simulink model "bsm1_ss_singlereactor"  (R2012b)
settings: Solver=ode45  SolverMode=SingleTasking  StartTime=0.0  StopTime=14  FixedStep=0.01  RelTol=1e-5  AbsTol=1e-8
values from neighbouring files (symbols this model uses):
  ACTIVATE = [ 0 ]    [init_bsm1.m]
  carb1 = 0    [reginit_bsm1.m]    (also in reginit_bsm1_2.m)
  KLa1 = 2    [reginit_bsm1.m]    (also in reginit_bsm1_2.m)
  TEMPMODEL = [ 0 ]    [init_bsm1.m]
undefined symbols (not defined in the file or in its folder): PAR1, SOSAT1, VOL1, XINIT1
settings Model: ExtModeTrigMode=oneshot  ExtModeArmWhenConnect=off  ExtModeAutoUpdateStatusClock=off  BufferReuse=off  Creator=ielulf  LastModifiedBy=lasn
settings DataIOCC: InitialState=xFinal  LimitDataPoints=off  SignalLoggingSaveFormat=ModelDataLogs  SaveOutput=off  TimeSaveName=t  SignalLoggingName=sigsOut  OutputOption=SpecifiedOutputTimes  OutputTimes=[0:(1/96):14]
settings OptimizationCC: BlockReduction=off  BooleanDataType=off  InlineInvariantSignals=on  OptimizeBlockIOStorage=off  BufferReuse=off  ExpressionFolding=off  LocalBlockOutputs=off  InitFltsAndDblsToZero=on
settings DebuggingCC: SaveWithParameterizedLinksMsg=none  SignalResolutionControl=TryResolveAllWithWarning  SolverPrmCheckMsg=none  InheritedTsInSrcMsg=none  MultiTaskDSMMsg=warning  MultiTaskCondExecSysMsg=none  FcnCallInpInsideContextMsg=UseLocalSettings  UnconnectedOutputMsg=none  StrictBusMsg=None
settings HardwareCC: TargetUnknown=on
settings RTWCC: TemplateMakefile=grt_unix.tmf  IncludeERTFirstTime=on
settings GRTTargetCC: TargetFcnLib=ansi_tfl_tmw.mat  CombineOutputUpdateFcns=off  GRTInterface=on

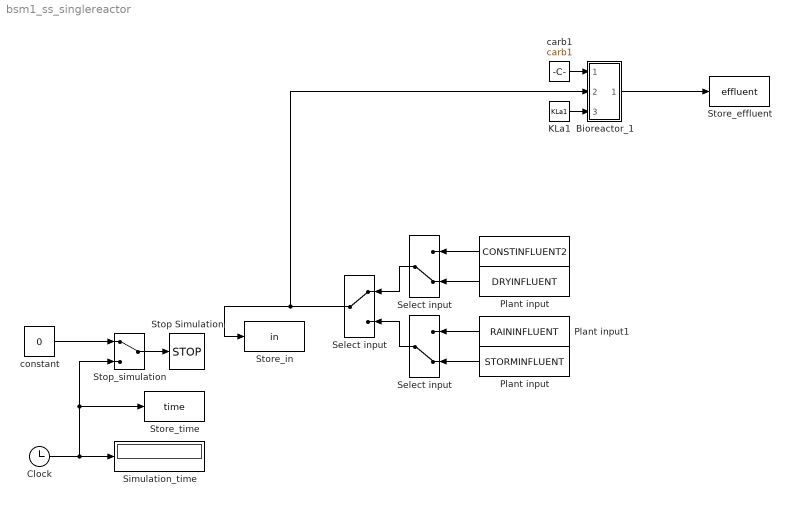
== system bsm1_ss_singlereactor ==
  " " : FromWorkspace  VariableName=CONSTINFLUENT2  OutputAfterFinalValue=Holding final value
  " Select input" : ManualSwitch
  " constant" : Constant  Value=0
  Bioreactor_1 : Subsystem
  Clock : Clock
  KLa1 : Constant  Value=KLa1
  Plant input : FromWorkspace  VariableName=DRYINFLUENT  OutputAfterFinalValue=Holding final value
  "Plant input " : FromWorkspace  VariableName=STORMINFLUENT  OutputAfterFinalValue=Holding final value
  Plant input1 : FromWorkspace  VariableName=RAININFLUENT  OutputAfterFinalValue=Holding final value
  Select input : ManualSwitch  CurrentSetting=0
  "Select input " : ManualSwitch  CurrentSetting=0
  Simulation_time : Display
  Stop Simulation : Stop
  Stop_simulation : ManualSwitch
  Store_effluent : ToWorkspace  VariableName=effluent
  Store_in : ToWorkspace  VariableName=in  SampleTime=-1
  Store_time : ToWorkspace  VariableName=time
  carb1 : Constant  Value=carb1
  wires:
  Clock/1 -> Simulation_time/1, Stop_simulation/2, Store_time/1
  Stop_simulation/1 -> Stop Simulation/1
  " constant"/1 -> Stop_simulation/1
  " Select input"/1 -> Bioreactor_1/2(in), Store_in/1
  KLa1/1 -> Bioreactor_1/3(KLa)
  carb1/1 -> Bioreactor_1/1(carb)
  Plant input/1 -> Select input/2
  " "/1 -> Select input/1
  Plant input1/1 -> "Select input "/1
  "Plant input "/1 -> "Select input "/2
  Select input/1 -> " Select input"/1
  "Select input "/1 -> " Select input"/2
  Bioreactor_1/1(out) -> Store_effluent/1

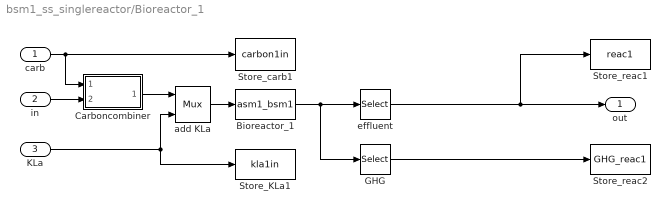
== system bsm1_ss_singlereactor/Bioreactor_1 ==
  carb : Inport
  in : Inport  Port=2
  KLa : Inport  Port=3
  Bioreactor_1 : S-Function  FunctionName=asm1_bsm1  Parameters=XINIT1,PAR1,VOL1,SOSAT1,TEMPMODEL,ACTIVATE  EnableBusSupport=off
  Carboncombiner : Subsystem
  GHG : Selector  InputPortWidth=29  IndexOptions=Index vector (dialog)  Indices=[27:29]  OutputSizes=1
  Store_KLa1 : ToWorkspace  VariableName=kla1in  SampleTime=-1
  Store_carb1 : ToWorkspace  VariableName=carbon1in  SampleTime=-1
  Store_reac1 : ToWorkspace  VariableName=reac1  SampleTime=-1
  Store_reac2 : ToWorkspace  VariableName=GHG_reac1  SampleTime=-1
  add KLa : Mux  Inputs=2
  effluent : Selector  InputPortWidth=29  IndexOptions=Index vector (dialog)  Indices=[1:26]  OutputSizes=1
  out : Outport
  wires:
  KLa/1 -> Store_KLa1/1, add KLa/2
  in/1 -> Carboncombiner/2(Input)
  carb/1 -> Carboncombiner/1(C_flow), Store_carb1/1
  Carboncombiner/1(Output) -> add KLa/1
  add KLa/1 -> Bioreactor_1/1
  Bioreactor_1/1 -> effluent/1, GHG/1
  effluent/1 -> out/1, Store_reac1/1
  GHG/1 -> Store_reac2/1

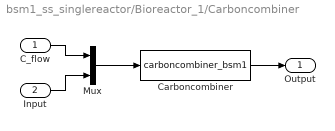
== system bsm1_ss_singlereactor/Bioreactor_1/Carboncombiner ==
  C_flow : Inport
  Input : Inport  Port=2
  Carboncombiner : S-Function  FunctionName=carboncombiner_bsm1  Parameters=CARBONSOURCECONC  EnableBusSupport=off
  Mux : Mux  Inputs=2
  Output : Outport
  wires:
  Input/1 -> Mux/2
  Carboncombiner/1 -> Output/1
  Mux/1 -> Carboncombiner/1
  C_flow/1 -> Mux/1
